simulink library "basic_THB"  (R2013b)
settings: Solver=ode45  StartTime=0.0  StopTime=10.0  RelTol=1e-3
settings Model: Creator=lena.frank  LastModifiedBy=drhf

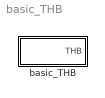
== system basic_THB ==
  basic_THB : Subsystem  mask(constant THV){t=20, mdot=0, p=1e5, ID=1, fluid=1, mix=0, mix2=0, mix3=0, dia=0.02, hgt=0}
      mask prompts: t "temperature [degree centigrade]"; mdot "massflow [kg/s]"; p "pressure [Pa]"; ID "Caclulation mode"; mix "fluid mixture [0..1]"; mix2 "fluid mixture 2 [0..1]"; mix3 "fluid mixture 3 [0..1]"; dia "diameter [m]"; hgt "Static height in m"
      mask help:
      | Create a constant Thermo-Hydraulic-Vector.
      | Calculation mode:
      |     1 ..  9999 no pressure drop (dp)
      | 10001 .. 19999 dp caused by flowrate
      | 20001 .. inf   dp by flowrate and static height
      mask init:
      | mix = min(1, max(0, mix));
      | dia = max(dia, 0.001);
      | ID = max(ID,1);
      mask Help: web(fullfile(path_carnot('help'),'basic_THB.html'),'-helpbrowser')

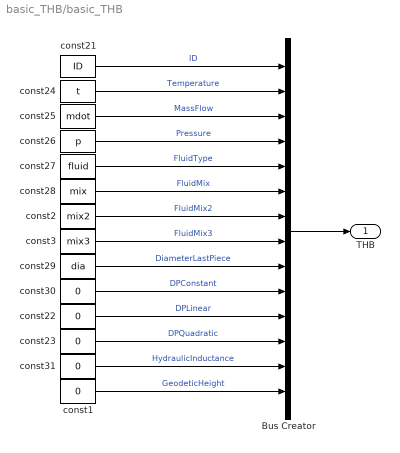
== system basic_THB/basic_THB ==
  Bus Creator : BusCreator  InitFcn=load THB.mat  Inputs=14  OutDataTypeStr=Bus: THB
  const{1,22..23,30..31} (5 alike) : Constant  Value=0
  const2 : Constant  Value=mix2
  const21 : Constant  Value=ID
  const24 : Constant  Value=t
  const25 : Constant  Value=mdot
  const26 : Constant  Value=p
  const27 : Constant  Value=fluid
  const28 : Constant  Value=mix
  const29 : Constant  Value=dia
  const3 : Constant  Value=mix3
  THB : Outport
  wires:
  const3/1 -> Bus Creator/8  "FluidMix3"
  const2/1 -> Bus Creator/7  "FluidMix2"
  const1/1 -> Bus Creator/14  "GeodeticHeight"
  const31/1 -> Bus Creator/13  "HydraulicInductance"
  const23/1 -> Bus Creator/12  "DPQuadratic"
  const22/1 -> Bus Creator/11  "DPLinear"
  const29/1 -> Bus Creator/9  "DiameterLastPiece"
  const30/1 -> Bus Creator/10  "DPConstant"
  Bus Creator/1 -> THB/1
  const21/1 -> Bus Creator/1  "ID"
  const24/1 -> Bus Creator/2  "Temperature"
  const25/1 -> Bus Creator/3  "MassFlow"
  const26/1 -> Bus Creator/4  "Pressure"
  const27/1 -> Bus Creator/5  "FluidType"
  const28/1 -> Bus Creator/6  "FluidMix"
